simulink model "s4"  (Simulink 2.00)
settings: Solver=ode15s  StartTime=0.0  StopTime=2.5  MaxStep=0.005  RelTol=1e-6  AbsTol=1e-6
values from neighbouring files (symbols this model uses):
  J = 0.8    [M1.M]    (also in M2.M = 2.5; M3A.M = 0.5; M3B.M = 0.5; M4.M = 0.015)
  Laq = 0.018    [M1.M]    (also in M2.M = 0.012; M3A.M; M3B.M; M4.M = 0.01)
  Lse = 0.026    [M4.M]    (also in M5.M = 0.044)
  Ra = 0.24    [M1.M]    (also in M2.M = 0.3; M3A.M = 0.14; M3B.M = 0.14; M4.M = 0.6)
  Rse = 0.1    [M4.M]    (also in M5.M = 0.2)
  SEIP4 = [-14.225 -12.275 -10.725 -9.725 -9.100 -8.600  -8.075 -7.650 -7.200 -6.850 -6.492 -6.135 -5.775 -5.112 -4.500  -3.825 -3.275 -2.783 -2.250 -1.688 -1.125 -0.542 0.0 0.542 1.125   1.688  2.250  2.783  3.275  3.825  4.500  5.112  5.775  6.135   6.492  6.850  7.200  7.650  8.075  8.600  9.100  9.725 10.725  12.275 14.225 ]    [M4.M]
  SEVP4 = [-160 -155 -150 -145 -140 -135 -130 -125 -120   -115 -110 -105 -100 -90 -80 -70 -60 -50 -40 -30 -20 -10 0  10 20 30 40 50 60 70 80 90 100 105 110 115 120 125 130 135  140 145 150 155 160]    [M4.M]
  Sw4AC = 0    [M4.M]
  wm0 = 350    [M4.M]
  wmo = 2000*(2*pi)/60    (= 209.439510239)    [M1.M]    (also in M4.M = 157.079632679; M5.M = 125.663706144)
settings Model: MaxOrder=3  SaveTime=off  SaveOutput=off  ConsistencyChecking=off

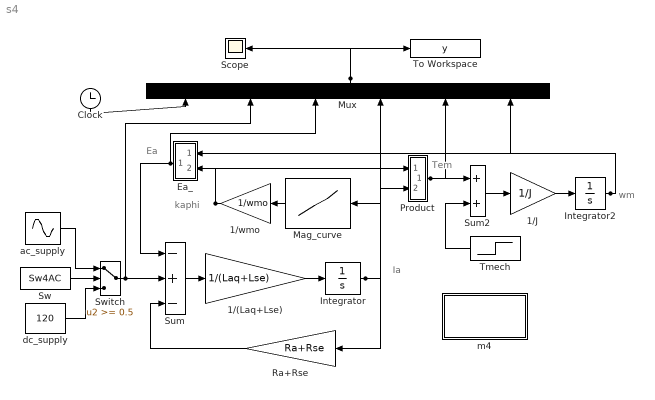
== system s4 ==
  note: wm
  note: Tem
  note: Ea
  note: kaphi
  note: Ia
  1/(Laq+Lse) : Gain  Gain=1/(Laq+Lse)
  1/J : Gain  Gain=1/J
  1/wmo : Gain  Orientation=left  Gain=1/wmo
  Clock : Clock
      settings: Orientation=down  DeleteFcn=simclock BlockIsBeingDestroyed  PostSaveFcn=simclock Save
  Ea_ : Subsystem  Orientation=left
      mask Type: Dot Product
      mask Description:
      | Inner (dot) product.
      | y=sum(u1.*u2)
      mask Help: Computes the inner (dot) product of the inputs: sum(u1.*u2).  The inputs are vectors of the same length. Output is a scalar.
      mask Display: disp('.\n')
  Integrator : Integrator  ExternalReset=none  InitialConditionSource=internal  InitialCondition=0  LimitOutput=off  UpperSaturationLimit=inf  LowerSaturationLimit=-inf  ShowSaturationPort=off  ShowStatePort=off  AbsoluteTolerance=auto
  Integrator2 : Integrator  ExternalReset=none  InitialConditionSource=internal  InitialCondition=wm0  LimitOutput=off  UpperSaturationLimit=inf  LowerSaturationLimit=-inf  ShowSaturationPort=off  ShowStatePort=off  AbsoluteTolerance=auto
  m4 : Subsystem
      settings: OpenFcn=m4
      mask Type: Masked block of m4.m
      mask Help: Uses m4.m to initialize and plot
      mask Display: disp('Initialize\nand plot')
  Mag_curve : Lookup  Orientation=left  InputValues=SEIP4  OutputValues=SEVP4
  Mux : Mux  Orientation=up  Inputs=6
  Product : Subsystem
      mask Type: Dot Product
      mask Description:
      | Inner (dot) product.
      | y=sum(u1.*u2)
      mask Help: Computes the inner (dot) product of the inputs: sum(u1.*u2).  The inputs are vectors of the same length. Output is a scalar.
      mask Display: disp('.\n')
  Ra+Rse : Gain  Orientation=left  Gain=Ra+Rse
  Scope : Scope
      settings: TickLabels=on  TimeRange=auto  YMin=-150  YMax=150  SaveToWorkspace=off  SaveName=ScopeData  LimitMaxRows=off
  Sum : Sum  Inputs=-+-
  Sum2 : Sum  Inputs=++
  Sw : Constant  Value=Sw4AC
  Switch : Switch  Threshold=0.5
  Tmech : Step  Orientation=left  Time=0.5  Before=-1  After=-0.5
  To Workspace : ToWorkspace  VariableName=y  SampleTime=0
      settings: Buffer=12000
  ac_supply : Sin  Amplitude=120*sqrt(2)  Frequency=377  Phase=0  SampleTime=-1
  dc_supply : Constant  Value=120
  wires:
  Switch/1 -> Mux/2, Sum/2
  Tmech/1 -> Sum2/2
  dc_supply/1 -> Switch/3
  Sw/1 -> Switch/2
  ac_supply/1 -> Switch/1
  Ea_/1(out_1) -> Mux/3, Sum/1
  Product/1(out_1) -> Mux/5, Sum2/1
  Integrator2/1 -> Mux/6, Ea_/1(in_1)
  Ra+Rse/1 -> Sum/3
  Integrator/1 -> Mag_curve/1, Mux/4, Product/2(in_2), Ra+Rse/1
  1/wmo/1 -> Ea_/2(in_2), Product/1(in_1)
  Mag_curve/1 -> 1/wmo/1
  Clock/1 -> Mux/1
  Mux/1 -> Scope/1, To Workspace/1
  1/(Laq+Lse)/1 -> Integrator/1
  1/J/1 -> Integrator2/1
  Sum2/1 -> 1/J/1
  Sum/1 -> 1/(Laq+Lse)/1

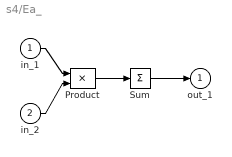
== system s4/Ea_ ==
  in_1 : Inport  Port=1  PortWidth=-1  SampleTime=-1
  in_2 : Inport  Port=2  PortWidth=-1  SampleTime=-1
  Product : Product  Inputs=2
  Sum : Sum  Inputs=+
  out_1 : Outport  Port=1  InitialOutput=0
  wires:
  Sum/1 -> out_1/1
  Product/1 -> Sum/1
  in_1/1 -> Product/1
  in_2/1 -> Product/2

== system s4/m4 ==
  note: Masked block of m4.m to initialize
      | s4.m in Chapter 8 and to plot results

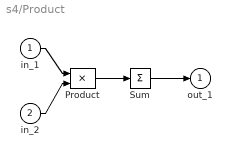
== system s4/Product ==
  in_1 : Inport  Port=1  PortWidth=-1  SampleTime=-1
  in_2 : Inport  Port=2  PortWidth=-1  SampleTime=-1
  Product : Product  Inputs=2
  Sum : Sum  Inputs=+
  out_1 : Outport  Port=1  InitialOutput=0
  wires:
  Sum/1 -> out_1/1
  Product/1 -> Sum/1
  in_1/1 -> Product/1
  in_2/1 -> Product/2
